simulink model "Final_EWASP_VC"  (R2022a)
settings: Solver=ode1  StartTime=0.0  StopTime=24*3600  FixedStep=10  RelTol=1e-3
values from neighbouring files (symbols this model uses):
  Aux_Threshold = 52    [Setup_Code_EWASP_VC.m]
  buildingAge = 2005    [Setup_Code_EWASP_VC.m]
  ceilingHeight = 2.4    [Setup_Code_EWASP_VC.m]
  conductiveHconnectMatrix = [ ... (first row only)    [Setup_Code_EWASP_VC.m]
  cRoofGreen = 100000    [Setup_Code_EWASP_VC.m]
  Defrost_After_Time = 30    [Setup_Code_EWASP_VC.m]
  DHWDemandProfile = occFreegainHotwaterElecTestPassiveOcc3(:,3)    [Setup_Code_EWASP_VC.m]
  Elec_Max = Elec_Max*(30/24.2)    [Setup_Code_EWASP_VC.m]
  Elec_Mid = Elec_Mid*(30/24.2)    [Setup_Code_EWASP_VC.m]
  Elec_Min = Elec_Min*(30/24.2)    [Setup_Code_EWASP_VC.m]
  ElecDemandProfile = occFreegainHotwaterElecTestPassiveOcc3(:,4)    [Setup_Code_EWASP_VC.m]
  ElecFixed = [Elec_Max(6,2) Elec_Max(6,4) Elec_Max(6,6) Elec_Max(6,7) ... (first row only)    [Setup_Code_EWASP_VC.m]
  floorOrCeilingArea = floorOrCeilingArea*1.15    [Setup_Code_EWASP_VC.m]
  forceCold = 0    [Setup_Code_EWASP_VC.m]
  freegain = occFreegainHotwaterElecTestPassiveOcc3(:,2)-max(occupancy)*25    [Setup_Code_EWASP_VC.m]
  furnitureModelOn = 1    [Setup_Code_EWASP_VC.m]
  Heat_Max = Heat_Max*(30/24.2)    [Setup_Code_EWASP_VC.m]
  Heat_Mid = Heat_Mid*(30/24.2)    [Setup_Code_EWASP_VC.m]
  Heat_Min = Heat_Min*(30/24.2)    [Setup_Code_EWASP_VC.m]
  HeatFixed = [Heat_Max(6,2) Heat_Max(6,4) Heat_Max(6,6) Heat_Max(6,7) ... (first row only)    [Setup_Code_EWASP_VC.m]
  HeatingOnProfile = repmat(HeatingOnProfile,365,1)    [Setup_Code_EWASP_VC.m]
  HEX_ReturnLowerLimit = 52.5    [Setup_Code_EWASP_VC.m]
  HEX_ReturnUpperLimit = 55    [Setup_Code_EWASP_VC.m]
  LeakMultiplier = 1+(2*(rand()-0.5)/10)    [Setup_Code_EWASP_VC.m]
  loopCap = 15    [Setup_Code_EWASP_VC.m]
  maxOcc = max(occupancyProfile)    [Setup_Code_EWASP_VC.m]
  NESW_wallArea = max(NESW_Lengths*ceilingHeight-NESW_Windows,0)    [Setup_Code_EWASP_VC.m]
  NESW_Windows = [ ... (first row only)    [Setup_Code_EWASP_VC.m]
  numRooms = roomCount    [Setup_Code_EWASP_VC.m]
  offsetDays = 0    [Setup_Code_EWASP_VC.m]
  pumpChoice = pumpChoices(MinIndex,1)    [Setup_Code_EWASP_VC.m]
  pumpRamp = 180    [Setup_Code_EWASP_VC.m]
  ReturnLowerLimit = 37.5    [Setup_Code_EWASP_VC.m]
  ReturnUpperLimit = 40    [Setup_Code_EWASP_VC.m]
  RoofIrradiance = Flat_NS_EW_RoofIrradiance(:,1)    [Setup_Code_EWASP_VC.m]
  roofStartTemp = ones(11,1)*20    [Setup_Code_EWASP_VC.m]
  rooftype = 0    [Setup_Code_EWASP_VC.m]
  RoomDataMatrix = [zeros(1,12);ones(1,12)*wallDensity;zeros(1,12);ones(1,12)*wallU;ones(1,12)*windowU;ones(1,12)*floorU;ones(1,12)*ceilingU;zeros(1,12);windowArea, 0;floorOrCeilingArea;zeros(1,12);floorOrCeilingArea*ceilingHeight]    [Setup_Code_EWASP_VC.m]
  roomVol = roomVol*1.15    [Setup_Code_EWASP_VC.m]
  slabStartTemp = (GroundTempTimeSeries(offsetDays*1440+1,1)+thermostatSetting)/2    [Setup_Code_EWASP_VC.m]
  SlackRequest = zeros(1440,1)    [Setup_Code_EWASP_VC.m]
  SolarThermalExists = 0    [Setup_Code_EWASP_VC.m]
  SourceFixed = HeatFixed-ElecFixed    [Setup_Code_EWASP_VC.m]
  StateSeries = StateSeriesGenerator(22,7,1)    [Setup_Code_EWASP_VC.m]
  Tank_Lower_Temp = 49.5    [Setup_Code_EWASP_VC.m]
  Tank_Upper_Temp = 52    [Setup_Code_EWASP_VC.m]
  Tank_Volume_m3 = 0.15    [Setup_Code_EWASP_VC.m]
  TankHeatHour = randi([1 5])-1    [Setup_Code_EWASP_VC.m]
  thermostatSetting = 20.0    (= 20)    [Setup_Code_EWASP_VC.m]
  upDown = [0;0;0;0;1;1;1;1;1;1;1]    [Setup_Code_EWASP_VC.m]
  variableASHP = 1    [Setup_Code_EWASP_VC.m]
  wallStartTempExt = thermostatSetting*(0.266+0.00215*outdoorStartTemp+0.018*wallU+0.00113*outdoorStartTemp*wallU+0.0068*wallU^2)    [Setup_Code_EWASP_VC.m]
undefined symbols (not defined in the file or in its folder): a, ceilingU, condUDMatrix, convUDMatrix, deltaPEXPANDED_E, deltaPEXPANDED_E2, deltaPEXPANDED_N, deltaPEXPANDED_N2, deltaPEXPANDED_S, deltaPEXPANDED_S2, deltaPEXPANDED_W, deltaPEXPANDED_W2, DesiredDHWTemp, DesiredFlowTempVsInOutDeltaTemp, DiffuseHorizontal, DiscIntNeverNeededParam, DNI, dwnAndConcrete, DWORK_A_HX, DWORK_CHK_FLU, DWORK_CP_NODE, DWORK_DH, DWORK_FLUID, DWORK_HCON, DWORK_LOSS, DWORK_MDOTDOWN, DWORK_MDOTIN, DWORK_MDOTUP, DWORK_MIX, DWORK_PRESS, DWORK_QDOTIN, DWORK_RHO_NODE, DWORK_TIN, DWORK_TS_OLD, DWORK_V_NODE, GroundTempTimeSeries, HCM, HCM2, HCM_closed, HCM_closed2, intermediateU, IsTop, massFlowMatrix, neighbourMatrix, numericalRoomUse, RadiatorMatrix, room2roomflowmatrix_E, room2roomflowmatrix_E2, room2roomflowmatrix_N, room2roomflowmatrix_N2, room2roomflowmatrix_S, room2roomflowmatrix_S2, room2roomflowmatrix_W, room2roomflowmatrix_W2, StateAirInEXPANDED_E, StateAirInEXPANDED_E2, StateAirInEXPANDED_N, StateAirInEXPANDED_N2, StateAirInEXPANDED_S, StateAirInEXPANDED_S2 ... (+23)
libraries: simulink x6, dspsigops x4, dspmtrx3 x4, carnot x3, spsEdgeDetectorLib x2, dspstat3 x2, powerlib_meascontrol x1, simulink_extras x1
(part 19 of 27)

== system Final_EWASP_VC/ASHP_Subsystem/DHW for ASHP Case/Storage_Type_2_CONF/Pipe_Connection_1 ==
  THBin : Inport
  Demux : Demux  Outputs=2
  Gain : Gain  Gain=in
  Gain1 : Gain  Gain=up
  Gain2 : Gain  Gain=down
  Gain3 : Gain  Gain=in
  Ground : Ground
  Ground1 : Ground
  Ground2 : Ground
  Mux3 : Mux  Inputs=8
  Q_in : Constant  Value=zeros(nodes,1)
  to_storeT : Outport  VectorParamsAs1DForOutWhenUnconnected=off
  wires:
  THBin/1 -> Demux/1
  Demux/2 -> Gain/1, Gain1/1, Gain2/1
  Demux/1 -> Gain3/1
  Gain/1 -> Mux3/2  "mdot_in"
  Gain1/1 -> Mux3/3  "mdot_up"
  Gain2/1 -> Mux3/4  "mdot_down"
  Mux3/1 -> to_storeT/1
  Gain3/1 -> Mux3/1  "T_in"
  Q_in/1 -> Mux3/5
  Ground/1 -> Mux3/6
  Ground1/1 -> Mux3/7
  Ground2/1 -> Mux3/8

== system Final_EWASP_VC/ASHP_Subsystem/DHW for ASHP Case/Storage_Type_2_CONF/Pipe_Connection_2 ==
  THBin : Inport
  Demux : Demux  Outputs=2
  Gain : Gain  Gain=in
  Gain1 : Gain  Gain=up
  Gain2 : Gain  Gain=down
  Gain3 : Gain  Gain=in
  Ground : Ground
  Ground1 : Ground
  Ground2 : Ground
  Mux3 : Mux  Inputs=8
  Q_in : Constant  Value=zeros(nodes,1)
  to_storeT : Outport  VectorParamsAs1DForOutWhenUnconnected=off
  wires:
  THBin/1 -> Demux/1
  Demux/2 -> Gain/1, Gain1/1, Gain2/1
  Gain2/1 -> Mux3/4  "mdot_down"
  Q_in/1 -> Mux3/5
  Gain1/1 -> Mux3/3  "mdot_up"
  Demux/1 -> Gain3/1
  Gain/1 -> Mux3/2  "mdot_in"
  Gain3/1 -> Mux3/1  "T_in"
  Mux3/1 -> to_storeT/1
  Ground2/1 -> Mux3/8
  Ground/1 -> Mux3/6
  Ground1/1 -> Mux3/7

== system Final_EWASP_VC/ASHP_Subsystem/Subsystem14/HeatPump_Simplified/HeatPump_basic ==
  Tin_cold : Inport
  Tin_hot : Inport  Port=2
  Tamb : Inport  Port=3
  Ctrl : Inport  Port=4
  mdot_in_cold : Inport  Port=5
  mdot_in_hot : Inport  Port=6
  Defrost Delta In : Inport  Port=7
  Ctrl1 : Inport  Port=8
  Bus Creator : BusCreator  Inputs=7
  P_el calculus : Subsystem
  Product : DotProduct  OutDataTypeStr=Inherit: Inherit via internal rule
  Product1 : DotProduct  OutDataTypeStr=Inherit: Inherit via internal rule
  Product3 : DotProduct  OutDataTypeStr=Inherit: Inherit via internal rule
  Sum1 : Sum  Inputs=+-  InputSameDT=on  SaturateOnIntegerOverflow=on  OutDataTypeStr=Inherit: Same as first input
  Sum2 : Sum  Inputs=+-  InputSameDT=on  SaturateOnIntegerOverflow=on  OutDataTypeStr=Inherit: Same as first input
  model cold side : Subsystem
  model hot side : Subsystem
  Tsource : Outport  VectorParamsAs1DForOutWhenUnconnected=off
  THBload : Outport  Port=2  VectorParamsAs1DForOutWhenUnconnected=off
  HPdat : Outport  Port=3  VectorParamsAs1DForOutWhenUnconnected=off
  Real P_Therm : Outport  Port=4  VectorParamsAs1DForOutWhenUnconnected=off
  Main Delta : Outport  Port=5  VectorParamsAs1DForOutWhenUnconnected=off
  wires:
  Bus Creator/1 -> HPdat/1
  model hot side/2(Thot_out) -> Bus Creator/5, THBload/1, model cold side/3(Thot), P_el calculus/1(Thot_out), Sum2/1  "Tout_hot"
  Tamb/1 -> model hot side/4(Tamb), model cold side/4(Tamb)
  Tin_hot/1 -> Bus Creator/4, Sum2/2, model hot side/2(Thot)  "THBin_hot"
  mdot_in_hot/1 -> model hot side/3(mdot_hot)
  model hot side/1(mdot*cp) -> Product/1
  Sum2/1 -> Product/2
  Tin_cold/1 -> Bus Creator/1, P_el calculus/2(Tcold_in), model hot side/1(Tcold), Sum1/1, model cold side/1(Tcold)
  model cold side/1(Tcold_out) -> Bus Creator/2, Tsource/1, Sum1/2  "Tcold_out"
  P_el calculus/1(P_el) -> Product1/2
  Product1/1 -> Bus Creator/7  "Pelec"
  Ctrl/1 -> model cold side/5(command), Product1/1, model hot side/5(command)
  mdot_in_cold/1 -> model cold side/2(mdot_cold)
  Sum1/1 -> Product3/1
  model cold side/2(mdot*cp) -> Product3/2
  Product3/1 -> Bus Creator/3  "Qdot_cold"
  Product/1 -> Bus Creator/6  "Qdot_hot"
  model hot side/3(Real P_therm) -> Real P_Therm/1
  model hot side/4(Main Delta) -> Main Delta/1
  Defrost Delta In/1 -> model hot side/6(Defrost Delta In)
  Ctrl1/1 -> model hot side/7(Tamb1)

== system Final_EWASP_VC/ASHP_Subsystem/Subsystem14/HeatPump_Simplified1/HeatPump_basic ==
  Tin_cold : Inport
  Tin_hot : Inport  Port=2
  Tamb : Inport  Port=3
  Ctrl : Inport  Port=4
  mdot_in_cold : Inport  Port=5
  mdot_in_hot : Inport  Port=6
  Main Delta In : Inport  Port=7
  Bus Creator : BusCreator  Inputs=7
  P_el calculus : Subsystem
  Product : DotProduct  OutDataTypeStr=Inherit: Inherit via internal rule
  Product1 : DotProduct  OutDataTypeStr=Inherit: Inherit via internal rule
  Product3 : DotProduct  OutDataTypeStr=Inherit: Inherit via internal rule
  Sum1 : Sum  Inputs=+-  InputSameDT=on  SaturateOnIntegerOverflow=on  OutDataTypeStr=Inherit: Same as first input
  Sum2 : Sum  Inputs=+-  InputSameDT=on  SaturateOnIntegerOverflow=on  OutDataTypeStr=Inherit: Same as first input
  model cold side : Subsystem
  model hot side : Subsystem
  Tsource : Outport  VectorParamsAs1DForOutWhenUnconnected=off
  THBload : Outport  Port=2  VectorParamsAs1DForOutWhenUnconnected=off
  HPdat : Outport  Port=3  VectorParamsAs1DForOutWhenUnconnected=off
  Real P_Therm : Outport  Port=4  VectorParamsAs1DForOutWhenUnconnected=off
  Defrost Delta : Outport  Port=5  VectorParamsAs1DForOutWhenUnconnected=off
  wires:
  Bus Creator/1 -> HPdat/1
  model hot side/2(Thot_out) -> Bus Creator/5, THBload/1, model cold side/3(Thot), P_el calculus/1(Thot_out), Sum2/1  "Tout_hot"
  Tamb/1 -> model hot side/4(Tamb), model cold side/4(Tamb)
  Tin_hot/1 -> Bus Creator/4, Sum2/2, model hot side/2(Thot)  "THBin_hot"
  mdot_in_hot/1 -> model hot side/3(mdot_hot)
  model hot side/1(mdot*cp) -> Product/1
  Sum2/1 -> Product/2
  Tin_cold/1 -> Bus Creator/1, P_el calculus/2(Tcold_in), model hot side/1(Tcold), Sum1/1, model cold side/1(Tcold)
  model cold side/1(Tcold_out) -> Bus Creator/2, Tsource/1, Sum1/2  "Tcold_out"
  P_el calculus/1(P_el) -> Product1/2
  Product1/1 -> Bus Creator/7  "Pelec"
  Ctrl/1 -> model cold side/5(command), Product1/1, model hot side/5(command)
  mdot_in_cold/1 -> model cold side/2(mdot_cold)
  Sum1/1 -> Product3/1
  model cold side/2(mdot*cp) -> Product3/2
  Product3/1 -> Bus Creator/3  "Qdot_cold"
  Product/1 -> Bus Creator/6  "Qdot_hot"
  model hot side/3(Real P_therm) -> Real P_Therm/1
  model hot side/4(Defrost Delta) -> Defrost Delta/1
  Main Delta In/1 -> model hot side/6(Main Delta In)

== system Final_EWASP_VC/ASHP_Subsystem_Variable/DHW for ASHP Case/HeatPump_Simplified1/HeatPump_basic ==
  Tin_cold : Inport
  Tin_hot : Inport  Port=2
  Tamb : Inport  Port=3
  Ctrl : Inport  Port=4
  mdot_in_cold : Inport  Port=5
  mdot_in_hot : Inport  Port=6
  Main Delta In : Inport  Port=7
  Bus Creator : BusCreator  Inputs=7
  P_el calculus : Subsystem
  Product : DotProduct  OutDataTypeStr=Inherit: Inherit via internal rule
  Product1 : DotProduct  OutDataTypeStr=Inherit: Inherit via internal rule
  Product3 : DotProduct  OutDataTypeStr=Inherit: Inherit via internal rule
  Sum1 : Sum  Inputs=+-  InputSameDT=on  SaturateOnIntegerOverflow=on  OutDataTypeStr=Inherit: Same as first input
  Sum2 : Sum  Inputs=+-  InputSameDT=on  SaturateOnIntegerOverflow=on  OutDataTypeStr=Inherit: Same as first input
  model cold side : Subsystem
  model hot side : Subsystem
  Tsource : Outport  VectorParamsAs1DForOutWhenUnconnected=off
  THBload : Outport  Port=2  VectorParamsAs1DForOutWhenUnconnected=off
  HPdat : Outport  Port=3  VectorParamsAs1DForOutWhenUnconnected=off
  Real P_Therm : Outport  Port=4  VectorParamsAs1DForOutWhenUnconnected=off
  Defrost Delta : Outport  Port=5  VectorParamsAs1DForOutWhenUnconnected=off
  wires:
  Bus Creator/1 -> HPdat/1
  model hot side/2(Thot_out) -> Bus Creator/5, THBload/1, model cold side/3(Thot), P_el calculus/1(Thot_out), Sum2/1  "Tout_hot"
  Tamb/1 -> model hot side/4(Tamb), model cold side/4(Tamb)
  Tin_hot/1 -> Bus Creator/4, Sum2/2, model hot side/2(Thot)  "THBin_hot"
  mdot_in_hot/1 -> model hot side/3(mdot_hot)
  model hot side/1(mdot*cp) -> Product/1
  Sum2/1 -> Product/2
  Tin_cold/1 -> Bus Creator/1, P_el calculus/2(Tcold_in), model hot side/1(Tcold), Sum1/1, model cold side/1(Tcold)
  model cold side/1(Tcold_out) -> Bus Creator/2, Tsource/1, Sum1/2  "Tcold_out"
  P_el calculus/1(P_el) -> Product1/2
  Product1/1 -> Bus Creator/7  "Pelec"
  Ctrl/1 -> model cold side/5(command), Product1/1, model hot side/5(command)
  mdot_in_cold/1 -> model cold side/2(mdot_cold)
  Sum1/1 -> Product3/1
  model cold side/2(mdot*cp) -> Product3/2
  Product3/1 -> Bus Creator/3  "Qdot_cold"
  Product/1 -> Bus Creator/6  "Qdot_hot"
  model hot side/3(Real P_therm) -> Real P_Therm/1
  model hot side/4(Defrost Delta) -> Defrost Delta/1
  Main Delta In/1 -> model hot side/6(Main Delta In)

== system Final_EWASP_VC/ASHP_Subsystem_Variable/DHW for ASHP Case/HeatPump_Simplified2/HeatPump_basic ==
  Tin_cold : Inport
  Tin_hot : Inport  Port=2
  Tamb : Inport  Port=3
  Ctrl : Inport  Port=4
  mdot_in_cold : Inport  Port=5
  mdot_in_hot : Inport  Port=6
  Defrost Delta In : Inport  Port=7
  Bus Creator : BusCreator  Inputs=7
  P_el calculus : Subsystem
  Product : DotProduct  OutDataTypeStr=Inherit: Inherit via internal rule
  Product1 : DotProduct  OutDataTypeStr=Inherit: Inherit via internal rule
  Product3 : DotProduct  OutDataTypeStr=Inherit: Inherit via internal rule
  Sum1 : Sum  Inputs=+-  InputSameDT=on  SaturateOnIntegerOverflow=on  OutDataTypeStr=Inherit: Same as first input
  Sum2 : Sum  Inputs=+-  InputSameDT=on  SaturateOnIntegerOverflow=on  OutDataTypeStr=Inherit: Same as first input
  model cold side : Subsystem
  model hot side : Subsystem
  Tsource : Outport  VectorParamsAs1DForOutWhenUnconnected=off
  THBload : Outport  Port=2  VectorParamsAs1DForOutWhenUnconnected=off
  HPdat : Outport  Port=3  VectorParamsAs1DForOutWhenUnconnected=off
  Real P_Therm : Outport  Port=4  VectorParamsAs1DForOutWhenUnconnected=off
  Main Delta : Outport  Port=5  VectorParamsAs1DForOutWhenUnconnected=off
  wires:
  Bus Creator/1 -> HPdat/1
  model hot side/2(Thot_out) -> Bus Creator/5, THBload/1, model cold side/3(Thot), P_el calculus/1(Thot_out), Sum2/1  "Tout_hot"
  Tamb/1 -> model hot side/4(Tamb), model cold side/4(Tamb)
  Tin_hot/1 -> Bus Creator/4, Sum2/2, model hot side/2(Thot)  "THBin_hot"
  mdot_in_hot/1 -> model hot side/3(mdot_hot)
  model hot side/1(mdot*cp) -> Product/1
  Sum2/1 -> Product/2
  Tin_cold/1 -> Bus Creator/1, P_el calculus/2(Tcold_in), model hot side/1(Tcold), Sum1/1, model cold side/1(Tcold)
  model cold side/1(Tcold_out) -> Bus Creator/2, Tsource/1, Sum1/2  "Tcold_out"
  P_el calculus/1(P_el) -> Product1/2
  Product1/1 -> Bus Creator/7  "Pelec"
  Ctrl/1 -> model cold side/5(command), Product1/1, model hot side/5(command)
  mdot_in_cold/1 -> model cold side/2(mdot_cold)
  Sum1/1 -> Product3/1
  model cold side/2(mdot*cp) -> Product3/2
  Product3/1 -> Bus Creator/3  "Qdot_cold"
  Product/1 -> Bus Creator/6  "Qdot_hot"
  model hot side/3(Real P_therm) -> Real P_Therm/1
  model hot side/4(Main Delta) -> Main Delta/1
  Defrost Delta In/1 -> model hot side/6(Defrost Delta In)

== system Final_EWASP_VC/ASHP_Subsystem_Variable/DHW for ASHP Case/Storage_Type_2_CONF/HX_EN12977_1 ==
  from_storeT : Inport
  Tempin : Inport  Port=2
  massFlowIn : Inport  Port=3
  Add1 : Sum  Inputs=+++
  C/C++ Code Block : S-Function  InitFcn=try, set_param(gcb,'FunctionName','selectHexOutTemp'), end  FunctionName=selectHexOutTemp  SFunctionModules=selectHexOutTemp_wrapper  SFunctionDeploymentMode=off  EnableBusSupport=off  mask(S-Function Builder){}
      mask help: Simulink:masks:SFunctionBuilder_MD
      mask init: same as Final_EWASP_VC/ASHP_Subsystem/DHW for ASHP Case/C/C++ Code Block
      settings: CopyFcn=set_param(gcbh,'LinkStatus','none')  PreSaveFcn=try, set_param(gcb,'FunctionName','selectHexOutTemp'), end  OpenFcn=sfunctionwizard(gcbh)
      mask Display: plot(val(:,1),val(:,2)),disp(sys), port_label('input',1,'u0'), port_label('output',1,'y0')
  Constant : Constant  Value=5000
  Constant1 : Constant  Value=0
  Demux1 : Demux  Outputs=10
  Mux1 : Mux  Inputs=10
  Mux3 : Mux  Inputs=8
  Scope : Scope
  Switch : Switch  Criteria=u2 > Threshold  SaturateOnIntegerOverflow=off  InputSameDT=off
  T_in : Constant  Value=zeros(nodes,1)
  fluid : Constant  Value=-9999
  mdot_in : Constant  Value=zeros(nodes,1)
  mix : Constant  Value=-9999
  p : Constant  Value=-9999
  sfun_storage_heatexchanger : Subsystem  AncestorBlock=carnot/Basic/Thermal_Models/sfun_storage_heatexchanger  mask(storage heat exchanger){idn=heat transfer data fit EN12977, nodes=nodes, inlet=inlet, outlet=outlet, p1=ua0, p2=uam, p3=uat, p4=0, p5=0, p6=0, p7=0}
      mask prompts: idn "type"; nodes "number of nodes"; inlet "inlet node"; outlet "outlet node"; p1 "Parameter 1"; p2 "Parameter 2"; p3 "Parameter 3"; p4 "Parameter 4"; p5 "Parameter 5"; p6 "Parameter 6"; p7 "Parameter 7"
      mask init: same as Final_EWASP_VC/ASHP_Subsystem/DHW for ASHP Case/Storage_Type_2_CONF/HX_EN12977_1/sfun_storage_heatexchanger
      mask Help: web(['file:///' fullfile(path_carnot('help'),'StoragePorts_HeatExchangerModels.html')],'-helpbrowser')
      mask TypeOptions idn: smooth tube theoretical | smooth tube theoretical - stratified | finned tube theoretical | finned tube theoretical  - stratified | heat transfer from data fit | heat transfer from data fit  - stratified | heat transfer data fit EN12977 | heat transfer data fit EN12977  - stratified
  to_storeT : Outport  VectorParamsAs1DForOutWhenUnconnected=off
  TempHEXout : Outport  Port=2  VectorParamsAs1DForOutWhenUnconnected=off
  AuxHeat : Outport  Port=3  VectorParamsAs1DForOutWhenUnconnected=off
  wires:
  mix/1 -> Mux3/8
  fluid/1 -> Mux3/7
  p/1 -> Mux3/6
  sfun_storage_heatexchanger/2(Thx) -> C/C++ Code Block/1, Scope/1
  sfun_storage_heatexchanger/1(Qnodes) -> Demux1/1  "Q_in"
  T_in/1 -> Mux3/1  "T_in"
  Mux3/1 -> to_storeT/1
  mdot_in/1 -> Mux3/4, Mux3/3, Mux3/2  "mdot_in"
  Tempin/1 -> sfun_storage_heatexchanger/2(Temperature)
  from_storeT/1 -> sfun_storage_heatexchanger/1(Tnodes)
  massFlowIn/1 -> sfun_storage_heatexchanger/3(MassFlow)
  C/C++ Code Block/1 -> TempHEXout/1
  Demux1/1 -> Add1/2
  Demux1/2 -> Mux1/2
  Demux1/3 -> Mux1/3
  Demux1/4 -> Mux1/4
  Demux1/8 -> Mux1/8
  Demux1/7 -> Mux1/7
  Demux1/5 -> Mux1/5
  Demux1/6 -> Mux1/6
  Demux1/10 -> Mux1/10
  Demux1/9 -> Mux1/9
  Add1/1 -> Mux1/1
  Switch/1 -> AuxHeat/1, Add1/1
  Constant/1 -> Switch/1
  Constant1/1 -> Switch/3
  [AuxOn] -> Switch/2
  Mux1/1 -> Mux3/5
  [SolarHeatToWater] -> Add1/3

== system Final_EWASP_VC/ASHP_Subsystem_Variable/DHW for ASHP Case/Storage_Type_2_CONF/Pipe_Connection_1 ==
  THBin : Inport
  Demux : Demux  Outputs=2
  Gain : Gain  Gain=in
  Gain1 : Gain  Gain=up
  Gain2 : Gain  Gain=down
  Gain3 : Gain  Gain=in
  Ground : Ground
  Ground1 : Ground
  Ground2 : Ground
  Mux3 : Mux  Inputs=8
  Q_in : Constant  Value=zeros(nodes,1)
  to_storeT : Outport  VectorParamsAs1DForOutWhenUnconnected=off
  wires:
  THBin/1 -> Demux/1
  Demux/2 -> Gain/1, Gain1/1, Gain2/1
  Demux/1 -> Gain3/1
  Gain/1 -> Mux3/2  "mdot_in"
  Gain1/1 -> Mux3/3  "mdot_up"
  Gain2/1 -> Mux3/4  "mdot_down"
  Mux3/1 -> to_storeT/1
  Gain3/1 -> Mux3/1  "T_in"
  Q_in/1 -> Mux3/5
  Ground/1 -> Mux3/6
  Ground1/1 -> Mux3/7
  Ground2/1 -> Mux3/8

== system Final_EWASP_VC/ASHP_Subsystem_Variable/DHW for ASHP Case/Storage_Type_2_CONF/Pipe_Connection_2 ==
  THBin : Inport
  Demux : Demux  Outputs=2
  Gain : Gain  Gain=in
  Gain1 : Gain  Gain=up
  Gain2 : Gain  Gain=down
  Gain3 : Gain  Gain=in
  Ground : Ground
  Ground1 : Ground
  Ground2 : Ground
  Mux3 : Mux  Inputs=8
  Q_in : Constant  Value=zeros(nodes,1)
  to_storeT : Outport  VectorParamsAs1DForOutWhenUnconnected=off
  wires:
  THBin/1 -> Demux/1
  Demux/2 -> Gain/1, Gain1/1, Gain2/1
  Gain2/1 -> Mux3/4  "mdot_down"
  Q_in/1 -> Mux3/5
  Gain1/1 -> Mux3/3  "mdot_up"
  Demux/1 -> Gain3/1
  Gain/1 -> Mux3/2  "mdot_in"
  Gain3/1 -> Mux3/1  "T_in"
  Mux3/1 -> to_storeT/1
  Ground2/1 -> Mux3/8
  Ground/1 -> Mux3/6
  Ground1/1 -> Mux3/7

== system Final_EWASP_VC/Airflow Model/Subsystem1/Subsystem/Determine flow in and flow out from net flow (+ve out, -ve in) ==
  In1 : Inport
  In2 : Inport  Port=2
  Minus{,2..3,5} (4 alike) : Sum  Inputs=+-
  Minus1 : Sum
  Minus4 : Sum
  Sum : Sum
  Sum1 : Sum
  Switch{,1..9} (10 alike) : Switch  Criteria=u2 > Threshold  SaturateOnIntegerOverflow=off  InputSameDT=off
  Unary Minus{,1..8} (9 alike) : UnaryMinus
  gradient multiplier : Lookup_n-D  NumberOfTableDimensions=1  BreakpointsForDimension1=[-5:5]  Table=|  InternalRulePriority=Speed  RndMeth=Simplest
      | flipud([0.17699115
      | 0.745098039
      | 0.316239316
      | 0.869565217
      | 0.451612903
      | 0
      | 0.548387097
      | 0.130434783
      | 0.683760684
      | 0.254901961
      | 0.82300885
      | ])
  gradient multiplier1 : Lookup_n-D  NumberOfTableDimensions=1  BreakpointsForDimension1=[-5:5]  Table=|  InternalRulePriority=Speed  RndMeth=Simplest
      | flipud([0.17699115
      | 0.745098039
      | 0.316239316
      | 0.869565217
      | 0.451612903
      | 0
      | 0.548387097
      | 0.130434783
      | 0.683760684
      | 0.254901961
      | 0.82300885
      | ])
  offsets : Lookup_n-D  NumberOfTableDimensions=1  BreakpointsForDimension1=[-5:5]  Table=|  InternalRulePriority=Speed  RndMeth=Simplest
      | ([0.08
      | 0.38
      | 0.185
      | 0.6
      | 0.42
      | 0
      | 0.51
      | 0.09
      | 0.4
      | 0.13
      | 0.372
      | ])
  offsets1 : Lookup_n-D  NumberOfTableDimensions=1  BreakpointsForDimension1=[-5:5]  Table=|  InternalRulePriority=Speed  RndMeth=Simplest
      | flipud([0.08
      | 0.38
      | 0.185
      | 0.6
      | 0.42
      | 0
      | 0.51
      | 0.09
      | 0.4
      | 0.13
      | 0.372
      | ])
  positive flow limit calc : Lookup_n-D  NumberOfTableDimensions=1  BreakpointsForDimension1=[-5:5]  Table=|  InternalRulePriority=Speed  RndMeth=Simplest
      | flipud([0.08
      | 0.38
      | 0.185
      | 0.6
      | 0.42
      | 0
      | 0.51
      | 0.09
      | 0.4
      | 0.13
      | 0.372])
  positive flow limit calc1 : Lookup_n-D  NumberOfTableDimensions=1  BreakpointsForDimension1=[-5:5]  Table=|  InternalRulePriority=Speed  RndMeth=Simplest
      | ([0.08
      | 0.38
      | 0.185
      | 0.6
      | 0.42
      | 0
      | 0.51
      | 0.09
      | 0.4
      | 0.13
      | 0.372])
  tempdiff : Constant  Value=3
  tempdiff{3..5,10..12} (6 alike) : Constant  Value=0
  tempdiff13 : Constant  Value=-1000
  tempdiff2 : Constant
  tempdiff6 : Constant  Value=1000
  tempdiff9 : Constant
  Out1 : Outport  VectorParamsAs1DForOutWhenUnconnected=off
  Out2 : Outport  Port=2  VectorParamsAs1DForOutWhenUnconnected=off
  wires:
  tempdiff12/1 -> Switch8/3
  tempdiff13/1 -> Switch7/3
  Unary Minus7/1 -> Minus5/2
  offsets1/1 -> Minus4/2
  Switch1/1 -> Minus2/1, Sum/1
  Switch9/1 -> Sum/2
  Switch2/1 -> Minus/1, Minus1/1
  gradient multiplier1/1 -> Switch6/1
  tempdiff9/1 -> Switch5/1
  positive flow limit calc1/1 -> Minus3/2
  Unary Minus/1 -> Switch/2
  Switch6/1 -> Minus5/1, Sum1/2
  Unary Minus5/1 -> Switch8/2
  tempdiff/1 -> offsets/1, positive flow limit calc/1
  Switch7/1 -> Unary Minus4/1, Unary Minus3/1
  Unary Minus1/1 -> Switch5/2
  tempdiff10/1 -> Switch5/3
  In1/1 -> Minus2/2, Switch4/2, Switch3/2, Switch3/1, Switch2/1, Switch2/2, Unary Minus6/1, Unary Minus8/1, Unary Minus7/1, Unary Minus5/1, Unary Minus2/1, Switch7/1
  Minus4/1 -> gradient multiplier1/1
  tempdiff11/1 -> Switch9/3
  Switch5/1 -> Switch6/2
  Switch/1 -> Switch1/2
  Switch8/1 -> Switch6/3
  Minus/1 -> Unary Minus/1
  Switch4/1 -> Sum1/1
  Minus5/1 -> Switch9/1
  In2/1 -> offsets1/1, positive flow limit calc1/1
  Minus3/1 -> Unary Minus1/1
  Unary Minus6/1 -> Switch8/1
  Unary Minus4/1 -> Minus4/1
  Unary Minus3/1 -> Minus3/1
  Unary Minus2/1 -> Switch7/2
  Minus2/1 -> Switch4/1
  Switch3/1 -> Switch1/3
  tempdiff5/1 -> Switch3/3
  offsets/1 -> Minus1/2
  tempdiff3/1 -> Switch/3
  Sum/1 -> Out2/1
  tempdiff6/1 -> Switch2/3
  tempdiff2/1 -> Switch/1
  gradient multiplier/1 -> Switch1/1
  Unary Minus8/1 -> Switch9/2
  tempdiff4/1 -> Switch4/3
  Sum1/1 -> Out1/1
  Minus1/1 -> gradient multiplier/1
  positive flow limit calc/1 -> Minus/2

== system Final_EWASP_VC/Airflow Model/Subsystem1/Subsystem/Subsystem ==
  In1 : Inport
  In2 : Inport  Port=2
  Extract Triangular Matrix : dspmtrx3/Extract Triangular Matrix  fcn=Upper  SimulateUsing=Code generation
      settings: SourceProductBaseCode=DS
  Extract Triangular Matrix1 : dspmtrx3/Extract Triangular Matrix  fcn=Upper  SimulateUsing=Code generation
      settings: SourceProductBaseCode=DS
  Plus : Sum
  Plus1 : Sum
  Transpose : Math  Operator=transpose  SignedPower=on
  Transpose1 : Math  Operator=transpose  SignedPower=on
  Out1 : Outport  VectorParamsAs1DForOutWhenUnconnected=off
  Out2 : Outport  Port=2  VectorParamsAs1DForOutWhenUnconnected=off
  wires:
  In1/1 -> Extract Triangular Matrix/1
  Transpose/1 -> Plus/1
  Extract Triangular Matrix1/1 -> Transpose1/1, Plus/2
  Extract Triangular Matrix/1 -> Plus1/1, Transpose/1
  In2/1 -> Extract Triangular Matrix1/1
  Transpose1/1 -> Plus1/2
  Plus1/1 -> Out1/1
  Plus/1 -> Out2/1

== system Final_EWASP_VC/Airflow Model/Subsystem1/Subsystem/Subsystem1 ==
  In1 : Inport
  Minus : Sum  Inputs=+-
  Minus1 : Sum  Inputs=+-
  Minus2 : Sum  Inputs=+-
  Selector : Selector  NumberOfDimensions=2  InputPortWidth=3  IndexOptions=Index vector (dialog),Index vector (dialog)  Indices=1:numRooms,1  OutputSizes=1,1
  Temp2density : MATLAB Function  TreatAsAtomicUnit=on
  Temp2density1 : MATLAB Function  TreatAsAtomicUnit=on
  Temp2density2 : MATLAB Function  TreatAsAtomicUnit=on
  average density of air between rooms represented by row and column : Subsystem
  deltaP(not height Corrected) between lower and upper2 : Constant  Value=upDown
  floorDensityCorrection : MATLAB Function  TreatAsAtomicUnit=on
  tempVector to average : MATLAB Function  TreatAsAtomicUnit=on
  tempVector to matrices : MATLAB Function  TreatAsAtomicUnit=on
  Out1 : Outport  VectorParamsAs1DForOutWhenUnconnected=off
  Out2 : Outport  Port=2  VectorParamsAs1DForOutWhenUnconnected=off
  wires:
  In1/1 -> tempVector to average/1(u), tempVector to matrices/1(u)
  Minus2/1 -> average density of air between rooms represented by row and column/2(In2), Minus/2
  tempVector to matrices/2(x) -> Temp2density/1(u)
  [floorCorrect] -> Minus2/2
  Minus1/1 -> Minus/1, average density of air between rooms represented by row and column/1(In1)
  tempVector to matrices/1(y) -> Temp2density1/1(u)
  Temp2density/1(y) -> Minus2/1
  [floorCorrect] -> Minus1/2
  Temp2density1/1(y) -> Minus1/1
  Minus/1 -> Out2/1
  average density of air between rooms represented by row and column/1(Out1) -> Out1/1
  Temp2density2/1(y) -> floorDensityCorrection/1(u)
  floorDensityCorrection/1(y) -> [floorCorrect]
  tempVector to average/1(y) -> floorDensityCorrection/3(w), Temp2density2/1(u)
  deltaP(not height Corrected) between lower and upper2/1 -> Selector/1
  Selector/1 -> floorDensityCorrection/2(v)

== system Final_EWASP_VC/Airflow Model/Subsystem2/Subsystem/Determine flow in and flow out from net flow (+ve out, -ve in) ==
  In1 : Inport
  In2 : Inport  Port=2
  Minus{,2..3,5} (4 alike) : Sum  Inputs=+-
  Minus1 : Sum
  Minus4 : Sum
  Scope1 : Scope
  Scope2 : Scope
  Scope3 : Scope
  Sum : Sum
  Sum of Elements1 : Sum  Inputs=+
  Sum of Elements4 : Sum  Inputs=+
  Sum1 : Sum
  Sum7 : Sum  Inputs=|-+
  Switch{,1..9} (10 alike) : Switch  Criteria=u2 > Threshold  SaturateOnIntegerOverflow=off  InputSameDT=off
  Unary Minus{,1..8} (9 alike) : UnaryMinus
  gradient multiplier : Lookup_n-D  NumberOfTableDimensions=1  BreakpointsForDimension1=[-5:5]  Table=|  InternalRulePriority=Speed  RndMeth=Simplest
      | flipud([0.17699115
      | 0.745098039
      | 0.316239316
      | 0.869565217
      | 0.451612903
      | 0
      | 0.548387097
      | 0.130434783
      | 0.683760684
      | 0.254901961
      | 0.82300885
      | ])
  gradient multiplier1 : Lookup_n-D  NumberOfTableDimensions=1  BreakpointsForDimension1=[-5:5]  Table=|  InternalRulePriority=Speed  RndMeth=Simplest
      | flipud([0.17699115
      | 0.745098039
      | 0.316239316
      | 0.869565217
      | 0.451612903
      | 0
      | 0.548387097
      | 0.130434783
      | 0.683760684
      | 0.254901961
      | 0.82300885
      | ])
  offsets : Lookup_n-D  NumberOfTableDimensions=1  BreakpointsForDimension1=[-5:5]  Table=|  InternalRulePriority=Speed  RndMeth=Simplest
      | ([0.08
      | 0.38
      | 0.185
      | 0.6
      | 0.42
      | 0
      | 0.51
      | 0.09
      | 0.4
      | 0.13
      | 0.372
      | ])
  offsets1 : Lookup_n-D  NumberOfTableDimensions=1  BreakpointsForDimension1=[-5:5]  Table=|  InternalRulePriority=Speed  RndMeth=Simplest
      | flipud([0.08
      | 0.38
      | 0.185
      | 0.6
      | 0.42
      | 0
      | 0.51
      | 0.09
      | 0.4
      | 0.13
      | 0.372
      | ])
  positive flow limit calc : Lookup_n-D  NumberOfTableDimensions=1  BreakpointsForDimension1=[-5:5]  Table=|  InternalRulePriority=Speed  RndMeth=Simplest
      | flipud([0.08
      | 0.38
      | 0.185
      | 0.6
      | 0.42
      | 0
      | 0.51
      | 0.09
      | 0.4
      | 0.13
      | 0.372])
  positive flow limit calc1 : Lookup_n-D  NumberOfTableDimensions=1  BreakpointsForDimension1=[-5:5]  Table=|  InternalRulePriority=Speed  RndMeth=Simplest
      | ([0.08
      | 0.38
      | 0.185
      | 0.6
      | 0.42
      | 0
      | 0.51
      | 0.09
      | 0.4
      | 0.13
      | 0.372])
  tempdiff : Constant  Value=3
  tempdiff{3..5,10..12} (6 alike) : Constant  Value=0
  tempdiff13 : Constant  Value=-1000
  tempdiff2 : Constant
  tempdiff6 : Constant  Value=1000
  tempdiff9 : Constant
  Out1 : Outport  VectorParamsAs1DForOutWhenUnconnected=off
  Out2 : Outport  Port=2  VectorParamsAs1DForOutWhenUnconnected=off
  wires:
  tempdiff12/1 -> Switch8/3
  tempdiff13/1 -> Switch7/3
  Unary Minus7/1 -> Minus5/2
  offsets1/1 -> Minus4/2
  Switch1/1 -> Minus2/1, Sum/1
  Switch9/1 -> Sum/2
  Switch2/1 -> Minus/1, Minus1/1
  gradient multiplier1/1 -> Switch6/1
  tempdiff9/1 -> Switch5/1
  positive flow limit calc1/1 -> Minus3/2
  Unary Minus/1 -> Switch/2
  Switch6/1 -> Minus5/1, Sum1/2
  Unary Minus5/1 -> Switch8/2
  tempdiff/1 -> offsets/1, positive flow limit calc/1
  Switch7/1 -> Unary Minus4/1, Unary Minus3/1
  Unary Minus1/1 -> Switch5/2
  tempdiff10/1 -> Switch5/3
  In1/1 -> Minus2/2, Switch4/2, Switch3/2, Switch3/1, Switch2/1, Switch2/2, Unary Minus6/1, Unary Minus8/1, Unary Minus7/1, Unary Minus5/1, Unary Minus2/1, Switch7/1
  Minus4/1 -> gradient multiplier1/1
  tempdiff11/1 -> Switch9/3
  Switch5/1 -> Switch6/2
  Switch/1 -> Switch1/2
  Switch8/1 -> Switch6/3
  Minus/1 -> Unary Minus/1
  Switch4/1 -> Sum1/1
  Minus5/1 -> Switch9/1
  In2/1 -> offsets1/1, positive flow limit calc1/1
  Minus3/1 -> Unary Minus1/1
  Unary Minus6/1 -> Switch8/1
  Unary Minus4/1 -> Minus4/1
  Unary Minus3/1 -> Minus3/1
  Unary Minus2/1 -> Switch7/2
  Minus2/1 -> Switch4/1
  Switch3/1 -> Switch1/3
  tempdiff5/1 -> Switch3/3
  offsets/1 -> Minus1/2
  tempdiff3/1 -> Switch/3
  tempdiff6/1 -> Switch2/3
  tempdiff2/1 -> Switch/1
  gradient multiplier/1 -> Switch1/1
  Unary Minus8/1 -> Switch9/2
  tempdiff4/1 -> Switch4/3
  Sum1/1 -> Sum of Elements4/1, Out1/1
  Minus1/1 -> gradient multiplier/1
  positive flow limit calc/1 -> Minus/2
  Sum of Elements4/1 -> Sum7/1, Scope2/1
  Sum/1 -> Sum of Elements1/1, Out2/1
  Sum of Elements1/1 -> Sum7/2, Scope1/1
  Sum7/1 -> Scope3/1

== system Final_EWASP_VC/Airflow Model/Subsystem2/Subsystem/Subsystem1 ==
  In1 : Inport
  Minus : Sum  Inputs=+-
  Minus1 : Sum  Inputs=+-
  Minus2 : Sum  Inputs=+-
  Selector : Selector  NumberOfDimensions=2  InputPortWidth=3  IndexOptions=Index vector (dialog),Index vector (dialog)  Indices=1:numRooms,1  OutputSizes=1,1
  Temp2density : MATLAB Function  TreatAsAtomicUnit=on
  Temp2density1 : MATLAB Function  TreatAsAtomicUnit=on
  Temp2density2 : MATLAB Function  TreatAsAtomicUnit=on
  average density of air between rooms represented by row and column : Subsystem
  deltaP(not height Corrected) between lower and upper2 : Constant  Value=upDown
  floorDensityCorrection : MATLAB Function  TreatAsAtomicUnit=on
  tempVector to average : MATLAB Function  TreatAsAtomicUnit=on
  tempVector to matrices : MATLAB Function  TreatAsAtomicUnit=on
  Out1 : Outport  VectorParamsAs1DForOutWhenUnconnected=off
  Out2 : Outport  Port=2  VectorParamsAs1DForOutWhenUnconnected=off
  wires:
  In1/1 -> tempVector to average/1(u), tempVector to matrices/1(u)
  Minus2/1 -> average density of air between rooms represented by row and column/2(In2), Minus/2
  tempVector to matrices/2(x) -> Temp2density/1(u)
  [floorCorrect] -> Minus2/2
  Minus1/1 -> Minus/1, average density of air between rooms represented by row and column/1(In1)
  tempVector to matrices/1(y) -> Temp2density1/1(u)
  Temp2density/1(y) -> Minus2/1
  [floorCorrect] -> Minus1/2
  Temp2density1/1(y) -> Minus1/1
  Minus/1 -> Out2/1
  average density of air between rooms represented by row and column/1(Out1) -> Out1/1
  Temp2density2/1(y) -> floorDensityCorrection/1(u)
  floorDensityCorrection/1(y) -> [floorCorrect]
  tempVector to average/1(y) -> floorDensityCorrection/3(w), Temp2density2/1(u)
  deltaP(not height Corrected) between lower and upper2/1 -> Selector/1
  Selector/1 -> floorDensityCorrection/2(v)

== system Final_EWASP_VC/Airflow Model/Subsystem2/Subsystem/Symmetry Mod ==
  In1 : Inport
  In2 : Inport  Port=2
  Extract Triangular Matrix : dspmtrx3/Extract Triangular Matrix  fcn=Upper  SimulateUsing=Code generation
      settings: SourceProductBaseCode=DS
  Extract Triangular Matrix1 : dspmtrx3/Extract Triangular Matrix  fcn=Upper  SimulateUsing=Code generation
      settings: SourceProductBaseCode=DS
  Plus : Sum
  Plus1 : Sum
  Transpose : Math  Operator=transpose  SignedPower=on
  Transpose1 : Math  Operator=transpose  SignedPower=on
  Out1 : Outport  VectorParamsAs1DForOutWhenUnconnected=off
  Out2 : Outport  Port=2  VectorParamsAs1DForOutWhenUnconnected=off
  wires:
  In1/1 -> Extract Triangular Matrix/1
  Transpose/1 -> Plus/1
  Extract Triangular Matrix1/1 -> Transpose1/1, Plus/2
  Extract Triangular Matrix/1 -> Plus1/1, Transpose/1
  In2/1 -> Extract Triangular Matrix1/1
  Transpose1/1 -> Plus1/2
  Plus1/1 -> Out1/1
  Plus/1 -> Out2/1

== system Final_EWASP_VC/GSHP_Subsystem/DHW for GSHP case/HeatPump_Simplified/HeatPump_basic ==
  Tin_cold : Inport
  Tin_hot : Inport  Port=2
  Tamb : Inport  Port=3
  Ctrl : Inport  Port=4
  mdot_in_cold : Inport  Port=5
  mdot_in_hot : Inport  Port=6
  Bus Creator : BusCreator  Inputs=7
  P_el calculus : Subsystem
  Product : DotProduct  OutDataTypeStr=Inherit: Inherit via internal rule
  Product1 : DotProduct  OutDataTypeStr=Inherit: Inherit via internal rule
  Product3 : DotProduct  OutDataTypeStr=Inherit: Inherit via internal rule
  Sum1 : Sum  Inputs=+-  InputSameDT=on  SaturateOnIntegerOverflow=on  OutDataTypeStr=Inherit: Same as first input
  Sum2 : Sum  Inputs=+-  InputSameDT=on  SaturateOnIntegerOverflow=on  OutDataTypeStr=Inherit: Same as first input
  model cold side : Subsystem
  model hot side : Subsystem
  Tsource : Outport  VectorParamsAs1DForOutWhenUnconnected=off
  THBload : Outport  Port=2  VectorParamsAs1DForOutWhenUnconnected=off
  HPdat : Outport  Port=3  VectorParamsAs1DForOutWhenUnconnected=off
  Real P_Therm : Outport  Port=4  VectorParamsAs1DForOutWhenUnconnected=off
  wires:
  Bus Creator/1 -> HPdat/1
  model hot side/2(Thot_out) -> Bus Creator/5, THBload/1, model cold side/3(Thot), P_el calculus/1(Thot_out), Sum2/1  "Tout_hot"
  Tamb/1 -> model hot side/4(Tamb), model cold side/4(Tamb)
  Tin_hot/1 -> Bus Creator/4, Sum2/2, model hot side/2(Thot)  "THBin_hot"
  mdot_in_hot/1 -> model hot side/3(mdot_hot)
  model hot side/1(mdot*cp) -> Product/1
  Sum2/1 -> Product/2
  Tin_cold/1 -> Bus Creator/1, P_el calculus/2(Tcold_in), model hot side/1(Tcold), Sum1/1, model cold side/1(Tcold)
  model cold side/1(Tcold_out) -> Bus Creator/2, Tsource/1, Sum1/2  "Tcold_out"
  P_el calculus/1(P_el) -> Product1/2
  Product1/1 -> Bus Creator/7  "Pelec"
  Ctrl/1 -> model cold side/5(command), Product1/1, model hot side/5(command)
  mdot_in_cold/1 -> model cold side/2(mdot_cold)
  Sum1/1 -> Product3/1
  model cold side/2(mdot*cp) -> Product3/2
  Product3/1 -> Bus Creator/3  "Qdot_cold"
  Product/1 -> Bus Creator/6  "Qdot_hot"
  model hot side/3(Real P_therm) -> Real P_Therm/1

== system Final_EWASP_VC/GSHP_Subsystem/DHW for GSHP case/Storage_Type_2_CONF/HX_EN12977_1 ==
  from_storeT : Inport
  Tempin : Inport  Port=2
  massFlowIn : Inport  Port=3
  Add1 : Sum  Inputs=+++
  C/C++ Code Block : S-Function  InitFcn=try, set_param(gcb,'FunctionName','selectHexOutTemp'), end  FunctionName=selectHexOutTemp  SFunctionModules=selectHexOutTemp_wrapper  SFunctionDeploymentMode=off  EnableBusSupport=off  mask(S-Function Builder){}
      mask help: Simulink:masks:SFunctionBuilder_MD
      mask init: same as Final_EWASP_VC/ASHP_Subsystem/DHW for ASHP Case/C/C++ Code Block
      settings: CopyFcn=set_param(gcbh,'LinkStatus','none')  PreSaveFcn=try, set_param(gcb,'FunctionName','selectHexOutTemp'), end  OpenFcn=sfunctionwizard(gcbh)
      mask Display: plot(val(:,1),val(:,2)),disp(sys), port_label('input',1,'u0'), port_label('output',1,'y0')
  Constant : Constant  Value=5000
  Constant1 : Constant  Value=0
  Demux1 : Demux  Outputs=10
  Mux1 : Mux  Inputs=10
  Mux3 : Mux  Inputs=8
  Scope : Scope
  Switch : Switch  Criteria=u2 > Threshold  SaturateOnIntegerOverflow=off  InputSameDT=off
  T_in : Constant  Value=zeros(nodes,1)
  fluid : Constant  Value=-9999
  mdot_in : Constant  Value=zeros(nodes,1)
  mix : Constant  Value=-9999
  p : Constant  Value=-9999
  sfun_storage_heatexchanger : Subsystem  AncestorBlock=carnot/Basic/Thermal_Models/sfun_storage_heatexchanger  mask(storage heat exchanger){idn=heat transfer data fit EN12977, nodes=nodes, inlet=inlet, outlet=outlet, p1=ua0, p2=uam, p3=uat, p4=0, p5=0, p6=0, p7=0}
      mask prompts: idn "type"; nodes "number of nodes"; inlet "inlet node"; outlet "outlet node"; p1 "Parameter 1"; p2 "Parameter 2"; p3 "Parameter 3"; p4 "Parameter 4"; p5 "Parameter 5"; p6 "Parameter 6"; p7 "Parameter 7"
      mask init: same as Final_EWASP_VC/ASHP_Subsystem/DHW for ASHP Case/Storage_Type_2_CONF/HX_EN12977_1/sfun_storage_heatexchanger
      mask Help: web(['file:///' fullfile(path_carnot('help'),'StoragePorts_HeatExchangerModels.html')],'-helpbrowser')
      mask TypeOptions idn: smooth tube theoretical | smooth tube theoretical - stratified | finned tube theoretical | finned tube theoretical  - stratified | heat transfer from data fit | heat transfer from data fit  - stratified | heat transfer data fit EN12977 | heat transfer data fit EN12977  - stratified
  to_storeT : Outport  VectorParamsAs1DForOutWhenUnconnected=off
  TempHEXout : Outport  Port=2  VectorParamsAs1DForOutWhenUnconnected=off
  AuxHeat : Outport  Port=3  VectorParamsAs1DForOutWhenUnconnected=off
  wires:
  mix/1 -> Mux3/8
  fluid/1 -> Mux3/7
  p/1 -> Mux3/6
  sfun_storage_heatexchanger/2(Thx) -> C/C++ Code Block/1, Scope/1
  sfun_storage_heatexchanger/1(Qnodes) -> Demux1/1  "Q_in"
  T_in/1 -> Mux3/1  "T_in"
  Mux3/1 -> to_storeT/1
  mdot_in/1 -> Mux3/4, Mux3/3, Mux3/2  "mdot_in"
  Tempin/1 -> sfun_storage_heatexchanger/2(Temperature)
  from_storeT/1 -> sfun_storage_heatexchanger/1(Tnodes)
  massFlowIn/1 -> sfun_storage_heatexchanger/3(MassFlow)
  C/C++ Code Block/1 -> TempHEXout/1
  Demux1/1 -> Add1/2
  Demux1/2 -> Mux1/2
  Demux1/3 -> Mux1/3
  Demux1/4 -> Mux1/4
  Demux1/8 -> Mux1/8
  Demux1/7 -> Mux1/7
  Demux1/5 -> Mux1/5
  Demux1/6 -> Mux1/6
  Demux1/10 -> Mux1/10
  Demux1/9 -> Mux1/9
  Add1/1 -> Mux1/1
  Switch/1 -> Add1/1, AuxHeat/1
  Constant/1 -> Switch/1
  Constant1/1 -> Switch/3
  [AuxOn] -> Switch/2
  Mux1/1 -> Mux3/5
  [SolarHeatToWater] -> Add1/3

== system Final_EWASP_VC/GSHP_Subsystem/DHW for GSHP case/Storage_Type_2_CONF/Pipe_Connection_1 ==
  THBin : Inport
  Demux : Demux  Outputs=2
  Gain : Gain  Gain=in
  Gain1 : Gain  Gain=up
  Gain2 : Gain  Gain=down
  Gain3 : Gain  Gain=in
  Ground : Ground
  Ground1 : Ground
  Ground2 : Ground
  Mux3 : Mux  Inputs=8
  Q_in : Constant  Value=zeros(nodes,1)
  to_storeT : Outport  VectorParamsAs1DForOutWhenUnconnected=off
  wires:
  THBin/1 -> Demux/1
  Demux/2 -> Gain/1, Gain1/1, Gain2/1
  Demux/1 -> Gain3/1
  Gain/1 -> Mux3/2  "mdot_in"
  Gain1/1 -> Mux3/3  "mdot_up"
  Gain2/1 -> Mux3/4  "mdot_down"
  Mux3/1 -> to_storeT/1
  Gain3/1 -> Mux3/1  "T_in"
  Q_in/1 -> Mux3/5
  Ground/1 -> Mux3/6
  Ground1/1 -> Mux3/7
  Ground2/1 -> Mux3/8

== system Final_EWASP_VC/GSHP_Subsystem/DHW for GSHP case/Storage_Type_2_CONF/Pipe_Connection_2 ==
  THBin : Inport
  Demux : Demux  Outputs=2
  Gain : Gain  Gain=in
  Gain1 : Gain  Gain=up
  Gain2 : Gain  Gain=down
  Gain3 : Gain  Gain=in
  Ground : Ground
  Ground1 : Ground
  Ground2 : Ground
  Mux3 : Mux  Inputs=8
  Q_in : Constant  Value=zeros(nodes,1)
  to_storeT : Outport  VectorParamsAs1DForOutWhenUnconnected=off
  wires:
  THBin/1 -> Demux/1
  Demux/2 -> Gain/1, Gain1/1, Gain2/1
  Gain2/1 -> Mux3/4  "mdot_down"
  Q_in/1 -> Mux3/5
  Gain1/1 -> Mux3/3  "mdot_up"
  Demux/1 -> Gain3/1
  Gain/1 -> Mux3/2  "mdot_in"
  Gain3/1 -> Mux3/1  "T_in"
  Mux3/1 -> to_storeT/1
  Ground2/1 -> Mux3/8
  Ground/1 -> Mux3/6
  Ground1/1 -> Mux3/7

== system Final_EWASP_VC/GSHP_Subsystem/Subsystem3/Ground_Source_Heat_Exchanger1/Randbedingung 1 ==
  note: Qdown,i
  note: Qup,i
  note: Qtot,i
  T_Up : Inport
  T_Down : Inport  Port=2
  T_Earth(i,1) : Inport  Port=3
  Gain1 : Gain  Gain=L1/(2)  SaturateOnIntegerOverflow=on  OutDataTypeStr=Inherit: Same as input  ParamDataTypeStr=Inherit: Same as input
  Gain2 : Gain  Gain=L1/(2)  SaturateOnIntegerOverflow=on  OutDataTypeStr=Inherit: Same as input  ParamDataTypeStr=Inherit: Same as input
  Gain3 : Gain  Gain=(1)/L1  SaturateOnIntegerOverflow=on  OutDataTypeStr=Inherit: Same as input  ParamDataTypeStr=Inherit: Same as input
  Sum3 : Sum  Inputs=|-+  InputSameDT=on  SaturateOnIntegerOverflow=on  OutDataTypeStr=Inherit: Same as first input
  Sum4 : Sum  Inputs=-+  InputSameDT=on  SaturateOnIntegerOverflow=on  OutDataTypeStr=Inherit: Same as first input
  Sum5 : Sum  Inputs=|++  InputSameDT=on  SaturateOnIntegerOverflow=on  OutDataTypeStr=Inherit: Same as first input
  Sum6 : Sum  Inputs=|-+  InputSameDT=on  SaturateOnIntegerOverflow=on  OutDataTypeStr=Inherit: Same as first input
  T_Earth(i,0) : Outport  VectorParamsAs1DForOutWhenUnconnected=off
  wires:
  Sum3/1 -> Gain1/1
  Sum4/1 -> Gain2/1
  Gain1/1 -> Sum5/1
  Gain2/1 -> Sum5/2
  Sum5/1 -> Gain3/1
  Gain3/1 -> Sum6/1
  T_Down/1 -> Sum3/1
  T_Up/1 -> Sum4/1
  T_Earth(i,1)/1 -> Sum3/2, Sum4/2, Sum6/2
  Sum6/1 -> T_Earth(i,0)/1

== system Final_EWASP_VC/GSHP_Subsystem/Subsystem3/Ground_Source_Heat_Exchanger1/Randbedingung 2 ==
  note: T_Earth(i,DimRad)
  note: DeltaT
  T_Earth(i,0) : Inport
  T_Earth(i,1) : Inport  Port=2
  Dd6 : Gain  Gain=c4  Multiplication=Matrix(K*u)  SaturateOnIntegerOverflow=on  OutDataTypeStr=Inherit: Same as input  ParamDataTypeStr=Inherit: Same as input
  Sum2 : Sum  Inputs=|+-  InputSameDT=on  SaturateOnIntegerOverflow=on  OutDataTypeStr=Inherit: Same as first input
  Sum3 : Sum  Inputs=+-  InputSameDT=on  SaturateOnIntegerOverflow=on  OutDataTypeStr=Inherit: Same as first input
  Tearth DimRad : Constant  Value=T_null  VectorParams1D=off
  g-function : Subsystem
  T_Earth(i,DimRad) Gew : Outport  VectorParamsAs1DForOutWhenUnconnected=off
  T_Earth(i,DimRad) : Outport  Port=2  VectorParamsAs1DForOutWhenUnconnected=off
  wires:
  Sum2/1 -> Dd6/1, T_Earth(i,DimRad)/1
  Tearth DimRad/1 -> Sum2/1
  T_Earth(i,1)/1 -> Sum3/1
  T_Earth(i,0)/1 -> Sum3/2
  Dd6/1 -> T_Earth(i,DimRad) Gew/1
  Sum3/1 -> g-function/1(T(i,1)-T(i,0))
  g-function/1(DeltaT) -> Sum2/2

== system Final_EWASP_VC/GSHP_Subsystem/Subsystem3/Ground_Source_Heat_Exchanger1/Tdown ==
  In1 : Inport
  A mult : Product  Multiplication=Matrix(*)  RndMeth=Zero
  A1 : From  TagVisibility=global
  B mult : Product  Multiplication=Matrix(*)  RndMeth=Zero
  C mult : Product  Multiplication=Matrix(*)  RndMeth=Zero
  D mult : Product  Multiplication=Matrix(*)  RndMeth=Zero
  Integrator : Integrator  InitialCondition=Tdown_0
  Selector1 : Selector  InputPortWidth=DimAxi/2  IndexOptions=Index vector (dialog)  Indices=1  OutputSizes=1
  Selector2 : Selector  InputPortWidth=DimAxi/2  IndexOptions=Index vector (dialog)  Indices=2  OutputSizes=1
  Sum1 : Sum  Inputs=|++
  Sum2 : Sum  Inputs=++|
  Out1 : Outport  VectorParamsAs1DForOutWhenUnconnected=off
  Out2 : Outport  Port=2  VectorParamsAs1DForOutWhenUnconnected=off
  Out3 : Outport  Port=3  VectorParamsAs1DForOutWhenUnconnected=off
  wires:
  Selector2/1 -> Out3/1
  Selector1/1 -> Out2/1
  [D] -> D mult/1
  [C] -> C mult/1
  A1/1 -> A mult/1
  [B] -> B mult/1
  A mult/1 -> Sum1/2
  Integrator/1 -> C mult/2, A mult/2  "X"
  Sum1/1 -> Integrator/1  "Xdot"
  B mult/1 -> Sum1/1
  C mult/1 -> Sum2/2
  D mult/1 -> Sum2/1
  In1/1 -> D mult/2, B mult/2
  Sum2/1 -> Out1/1, Selector1/1, Selector2/1  "y"

== system Final_EWASP_VC/GSHP_Subsystem/Subsystem3/Ground_Source_Heat_Exchanger1/Tup ==
  In1 : Inport
  A mult : Product  Multiplication=Matrix(*)  RndMeth=Zero
  B mult : Product  Multiplication=Matrix(*)  RndMeth=Zero
  C mult : Product  Multiplication=Matrix(*)  RndMeth=Zero
  D mult : Product  Multiplication=Matrix(*)  RndMeth=Zero
  Integrator : Integrator  InitialCondition=Tup_0
  Selector1 : Selector  InputPortWidth=DimAxi/2  IndexOptions=Index vector (dialog)  Indices=1  OutputSizes=1
  Selector2 : Selector  InputPortWidth=DimAxi/2  IndexOptions=Index vector (dialog)  Indices=2  OutputSizes=1
  Sum1 : Sum  Inputs=|++
  Sum2 : Sum  Inputs=++|
  Out1 : Outport  VectorParamsAs1DForOutWhenUnconnected=off
  Out2 : Outport  Port=2  VectorParamsAs1DForOutWhenUnconnected=off
  Out3 : Outport  Port=3  VectorParamsAs1DForOutWhenUnconnected=off
  wires:
  Selector2/1 -> Out3/1
  Selector1/1 -> Out2/1
  [Du] -> D mult/1
  [Cu] -> C mult/1
  [Au] -> A mult/1
  [Bu] -> B mult/1
  A mult/1 -> Sum1/2
  Integrator/1 -> C mult/2, A mult/2  "X"
  Sum1/1 -> Integrator/1  "Xdot"
  B mult/1 -> Sum1/1
  C mult/1 -> Sum2/2
  D mult/1 -> Sum2/1
  In1/1 -> D mult/2, B mult/2
  Sum2/1 -> Out1/1, Selector1/1, Selector2/1  "y"

== system Final_EWASP_VC/GSHP_Subsystem/Subsystem3/Ground_Source_Heat_Exchanger1/mdot>0 ==
  In1 : Inport
  mdot : Inport  Port=2
  In4 : Inport  Port=3
  Add : Sum
  Fcn2 : Fcn  Expr=u>0
  Fcn3 : Fcn  Expr=u==0
  Product : Product  RndMeth=Zero
  Product1 : Product  RndMeth=Zero
  Out1 : Outport  VectorParamsAs1DForOutWhenUnconnected=off
  wires:
  Fcn3/1 -> Product1/1
  Fcn2/1 -> Product/2
  mdot/1 -> Fcn3/1, Fcn2/1
  In4/1 -> Product1/2
  Add/1 -> Out1/1
  In1/1 -> Product/1
  Product1/1 -> Add/2
  Product/1 -> Add/1

== system Final_EWASP_VC/GSHP_Subsystem/Subsystem3/Ground_Source_Heat_Exchanger1/mdot>1 ==
  In1 : Inport
  mdot : Inport  Port=2
  In4 : Inport  Port=3
  Add : Sum
  Fcn2 : Fcn  Expr=u>0
  Fcn3 : Fcn  Expr=u==0
  Product : Product  RndMeth=Zero
  Product1 : Product  RndMeth=Zero
  Out1 : Outport  VectorParamsAs1DForOutWhenUnconnected=off
  wires:
  Fcn3/1 -> Product1/1
  Fcn2/1 -> Product/2
  mdot/1 -> Fcn3/1, Fcn2/1
  In4/1 -> Product1/2
  Add/1 -> Out1/1
  In1/1 -> Product/1
  Product1/1 -> Add/2
  Product/1 -> Add/1

== system Final_EWASP_VC/GSHP_Subsystem/Subsystem3/Ground_Source_Heat_Exchanger1/mdot>2 ==
  In1 : Inport
  mdot : Inport  Port=2
  In4 : Inport  Port=3
  Add : Sum
  Fcn2 : Fcn  Expr=u>0
  Fcn3 : Fcn  Expr=u==0
  Product : Product  RndMeth=Zero
  Product1 : Product  RndMeth=Zero
  Out1 : Outport  VectorParamsAs1DForOutWhenUnconnected=off
  wires:
  Fcn3/1 -> Product1/1
  Fcn2/1 -> Product/2
  mdot/1 -> Fcn3/1, Fcn2/1
  In4/1 -> Product1/2
  Add/1 -> Out1/1
  In1/1 -> Product/1
  Product1/1 -> Add/2
  Product/1 -> Add/1

== system Final_EWASP_VC/GSHP_Subsystem/Subsystem3/Ground_Source_Heat_Exchanger1/mdot>3 ==
  In1 : Inport
  mdot : Inport  Port=2
  In4 : Inport  Port=3
  Add : Sum
  Fcn2 : Fcn  Expr=u>0
  Fcn3 : Fcn  Expr=u==0
  Product : Product  RndMeth=Zero
  Product1 : Product  RndMeth=Zero
  Out1 : Outport  VectorParamsAs1DForOutWhenUnconnected=off
  wires:
  Fcn3/1 -> Product1/1
  Fcn2/1 -> Product/2
  mdot/1 -> Fcn3/1, Fcn2/1
  In4/1 -> Product1/2
  Add/1 -> Out1/1
  In1/1 -> Product/1
  Product1/1 -> Add/2
  Product/1 -> Add/1

== system Final_EWASP_VC/GSHP_Subsystem/Subsystem3/Ground_Source_Heat_Exchanger1/mdot>4 ==
  In1 : Inport
  mdot : Inport  Port=2
  In4 : Inport  Port=3
  Add : Sum
  Fcn2 : Fcn  Expr=u>0
  Fcn3 : Fcn  Expr=u==0
  Product : Product  RndMeth=Zero
  Product1 : Product  RndMeth=Zero
  Out1 : Outport  VectorParamsAs1DForOutWhenUnconnected=off
  wires:
  Fcn3/1 -> Product1/1
  Fcn2/1 -> Product/2
  mdot/1 -> Fcn3/1, Fcn2/1
  In4/1 -> Product1/2
  Add/1 -> Out1/1
  In1/1 -> Product/1
  Product1/1 -> Add/2
  Product/1 -> Add/1
